simulink model "kelvin_voigt_1d"  (R2022b)
settings: Solver=VariableStepAuto  StartTime=0.0  StopTime=10  RelTol=1e-3
libraries: simulink_extras x1
settings Model: Creator=parth  LastModifiedBy=parth

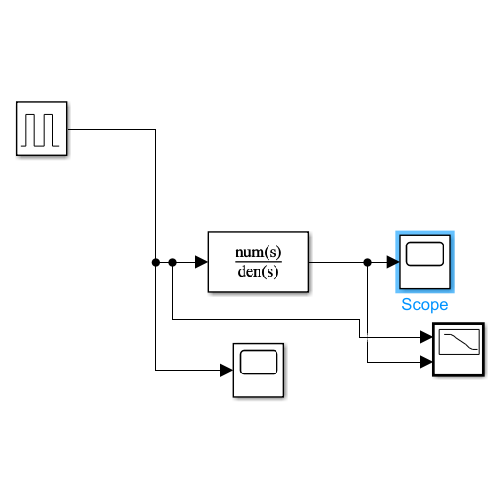
[thumbnail: Simulink's stored preview of the top-level diagram]
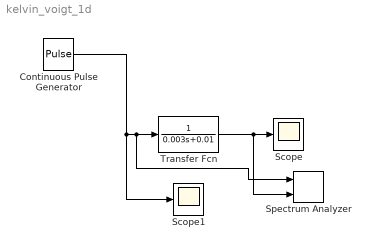
== system kelvin_voigt_1d ==
  Continuous Pulse Generator : DiscretePulseGenerator  PulseType=Time based  Period=1  PulseWidth=50
  Scope : Scope
  Scope1 : Scope
  Spectrum Analyzer : simulink_extras/Additional Sinks/Spectrum Analyzer  npts=256  fftpts=256  HowOften=64  sampleT=0.1
  Transfer Fcn : TransferFcn  Denominator=[0.003 0.01]
  wires:
  Transfer Fcn/1 -> Spectrum Analyzer/2, Scope/1
  Continuous Pulse Generator/1 -> Scope1/1, Spectrum Analyzer/1, Transfer Fcn/1
